simulink model "LeftCameraAgent"  (Simulink 6.2)
settings: Solver=ode45  StartTime=0.0  StopTime=10.0  RelTol=1e-3
settings Model: LastModifiedBy=suarezjl
settings DataIOCC: SignalLoggingName=sigsOut
settings HardwareCC: TargetUnknown=on

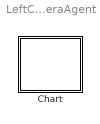
== system LeftCameraAgent ==
  Chart : Stateflow chart

== stateflow chart Chart ==
  state Initial
    \\Sally\CogDemo\HeadModule\LeftCameraAgent\FrameGrabber.Initialize()
    \\Sally\CogDemo\HeadModule\LeftCameraAgent\FrameGrabber.ObtainImage()
    \\Sally\CogDemo\HeadModule\LeftCameraAgent\FrameGrabber.ObtainImage()
    \\Sally\CogDemo\HeadModule\LeftCameraAgent\ColorBarney.Initialize()
    \\Sally\CogDemo\HeadModule\LeftCameraAgent\ColorBarney.LoadColorModel()
    \\Sally\CogDemo\HeadModule\LeftCameraAgent\ColorBlue.Initialize()
    \\Sally\CogDemo\HeadModule\LeftCameraAgent\ColorBlue.LoadColorModel()
    \\Sally\CogDemo\HeadModule\LeftCameraAgent\ColorRed.Initialize()
    \\Sally\CogDemo\HeadModule\LeftCameraAgent\ColorRed.LoadColorModel()
  state Segmentation
    \\Sally\CogDemo\HeadModule\LeftCameraAgent\FrameGrabber.ObtainImage()
    \\Sally\CogDemo\HeadModule\LeftCameraAgent\ColorBarney.DoSegment()
    \\Sally\CogDemo\HeadModule\LeftCameraAgent\ColorBlue.DoSegment()
    \\Sally\CogDemo\HeadModule\LeftCameraAgent\ColorRed.DoSegment()
  (default) -> Initial : Start
  Initial -> Segmentation : Always
  Segmentation -> Segmentation : Always
